simulink model "MotorDC_2"  (R2023a)
settings: Solver=VariableStepAuto  StartTime=0.0  StopTime=50  RelTol=1e-3
libraries: fl_lib x5, nesl_utility x5, ee_lib x1
settings Model: Creator=alexa  LastModifiedBy=alexa

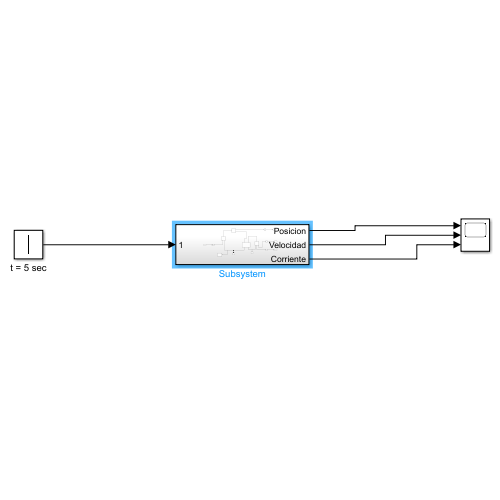
[thumbnail: Simulink's stored preview of the top-level diagram]
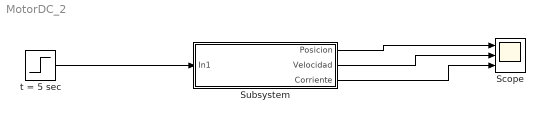
== system MotorDC_2 ==
  Scope : Scope  NumInputPorts=3
  Subsystem : Subsystem
  t = 5 sec : Step  Time=5  After=10.18  SampleTime=0
  wires:
  Subsystem/1(Posicion) -> Scope/1
  Subsystem/2(Velocidad) -> Scope/2
  t = 5 sec/1 -> Subsystem/1(In1)
  Subsystem/3(Corriente) -> Scope/3

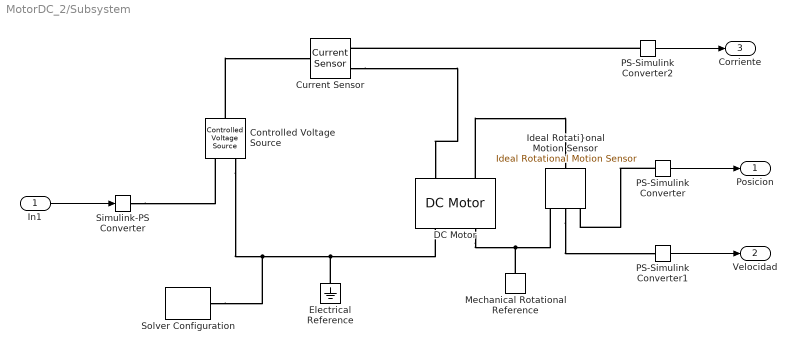
== system MotorDC_2/Subsystem ==
  In1 : Inport
  "Controlled Voltage Source " : fl_lib/Electrical/Electrical Sources/Controlled Voltage Source
  "Current Sensor " : fl_lib/Electrical/Electrical Sensors/Current Sensor
  "DC Motor " : ee_lib/Electromechanical/Brushed Motors/DC Motor  field_option=ee.enum.field_option.pm  Rf=100 Ohm  Lf=1 H  Laf=0.15 H  If0=0 A  parameterization=ee.enum.dcparam_option.circuit_param  Ra=7.61 Ohm  La=3.93e-3 H  emf_or_torque=ee.enum.emf_or_torque.ki  Kv=0.072e-3 V/rpm  Ki=2.17e-2 N*m/A  T_stall=0.24e-3 N*m  w_max=19100 rpm  w_rated=15000 rpm  P_rated=0.08 W  V_rated=1.5 V  lam_param=ee.enum.lam_param.damping  i_noload=0 A  V_i_noload=1.5 V  J=6.2e-5 kg*m^2  lam=5.98e-7 N*m*s/rad  speed0=0 rpm  enable_fault_armature=simscape.enum.onoff.off  rev_faulted=1 / 3  G_faulted_armature=1e-5 S  fault_trigger_armature=ee.enum.faults.faultTrigger.temporal  t_fault_armature=1 s  max_permissible_current_armature=inf A  t_fail_on_current_armature=1 s  enable_fault_field=simscape.enum.onoff.off  G_faulted_field=1e-5 S  fault_trigger_field=ee.enum.faults.faultTrigger.temporal  t_fault_field=1 s  max_permissible_current_field=inf A  t_fail_on_current_field=1 s  fault_action=simscape.enum.assert.action.none  alpha=3.93e-3 1/K  Tmeas=25 degC  thermal_mass=100 J/K  initial_temperature=25 degC
  Electrical Reference : fl_lib/Electrical/Electrical Elements/Electrical Reference
  "Ideal Rotati}onal Motion Sensor" : fl_lib/Mechanical/Mechanical Sensors/Ideal Rotational Motion Sensor  reference=foundation.enum.MeasurementReference.difference  acceleration_port=false  velocity_port=true  position_port=true  wrap_angle=false  offset=0 deg
  Mechanical Rotational Reference : fl_lib/Mechanical/Rotational Elements/Mechanical Rotational Reference
  PS-Simulink Converter : nesl_utility/PS-Simulink Converter  PhysicalDomain=network_engine_domain  SubClassName=ps_output  LeftPortType=input  RightPortType=output  PseudoPeriodic=off  Frequencies=[]  VectorFormat=inherit  Unit=inherit  AffineConversion=off
  PS-Simulink Converter1 : nesl_utility/PS-Simulink Converter  PhysicalDomain=network_engine_domain  SubClassName=ps_output  LeftPortType=input  RightPortType=output  PseudoPeriodic=off  Frequencies=[]  VectorFormat=inherit  Unit=inherit  AffineConversion=off
  "PS-Simulink Converter2 " : nesl_utility/PS-Simulink Converter  PhysicalDomain=network_engine_domain  SubClassName=ps_output  LeftPortType=input  RightPortType=output  PseudoPeriodic=off  Frequencies=[]  VectorFormat=inherit  Unit=inherit  AffineConversion=off
  Simulink-PS Converter : nesl_utility/Simulink-PS Converter  PhysicalDomain=network_engine_domain  SubClassName=ps_input  LeftPortType=input  RightPortType=output  PseudoPeriodic=off  Frequencies=[]  NoiseDistribution=none  NoiseParameters=[]  Unit=1  AffineConversion=off  FilteringAndDerivatives=provide  SimscapeFilterOrder=1  InputFilterTimeConstant=0.001  UdotUserProvided=0
  "Solver Configuration " : nesl_utility/Solver Configuration  PhysicalDomain=network_engine_domain  SubClassName=solver  LeftPortType=input  RightPortType=generic  Tones=[]  Harmonics=[]  SimulateNoise=off  Profile=off  UseLocalSampling=off  EnableSwitchedLinearOptims=on  FrequencyDomain=off  UseCCode=off  RelTol=0.001  AbsTol=0.001  MinStep=1e-09  ToWorkspace=off  RevertToSquareIcSolve=off  NumHomotopyIterations=100  PhasorMode=off  PhasorModeNumHarmonics=1  ConsistencySolver=NEWTON_XTOL_AFTER_FTOL  IndexReductionMethod=DerivativeReplacement  DoDC=off  ResidualTolerance=1e-09  ConsistencyTolSource=GLOBAL  ConsistencyAbsTol=0.001  ConsistencyRelTol=0.001  ConsistencyTolFactor=0.001  UseLocalSolver=off  LocalSolverChoice=NE_BACKWARD_EULER_ADVANCER  ResolveIndetEquations=on  FunctionEvalNumThread=1  LocalSolverSampleTime=0.001  DoFixedCost=off  MaxNonlinIter=3  MaxModeIter=2  ComputeImpulses=off  ImpulseIterations=2  LinearAlgebra=auto  LinearAlgebraNumThread=0  EquationFormulation=NE_TIME_EF  DelaysMemoryBudget=1024  AutomaticFiltering=on  FilteringTimeConstant=0.001  PartitionStorageMethod=AS_NEEDED  PartitionMemoryBudget=1024  PartitionMethod=ROBUST
  Posicion : Outport
  Velocidad : Outport  Port=2
  Corriente : Outport  Port=3
  wires:
  In1/1 -> Simulink-PS Converter/1
  PS-Simulink Converter/1 -> Posicion/1
  PS-Simulink Converter1/1 -> Velocidad/1
  "PS-Simulink Converter2 "/1 -> Corriente/1
  connections:
  "Controlled Voltage Source "/RConn2 -- "Solver Configuration "/RConn1 -- Electrical Reference/LConn1 -- "DC Motor "/RConn1
  "DC Motor "/LConn2 -- "Ideal Rotati}onal Motion Sensor"/LConn1
  "DC Motor "/RConn2 -- Mechanical Rotational Reference/LConn1 -- "Ideal Rotati}onal Motion Sensor"/RConn1
  Simulink-PS Converter/RConn1 -- "Controlled Voltage Source "/RConn1
  "Ideal Rotati}onal Motion Sensor"/RConn2 -- PS-Simulink Converter1/LConn1
  "PS-Simulink Converter2 "/LConn1 -- "Current Sensor "/RConn1
  "Current Sensor "/RConn2 -- "DC Motor "/LConn1
  PS-Simulink Converter/LConn1 -- "Ideal Rotati}onal Motion Sensor"/RConn3
  "Controlled Voltage Source "/LConn1 -- "Current Sensor "/LConn1
